simulink model "RT_TestMV_ATS"  (R2015b)
settings: Solver=FixedStepDiscrete  StartTime=0.0  StopTime=44.14  FixedStep=samplePeriod  RelTol=1e-3
PreLoadFcn:
  | initialize;
  | scramInitialize;
  | KR_alpha;
  | Discrete_Compensator;
  | ATS_setup
values from neighbouring files (symbols this model uses):
  a_ratio = K2/K1    (= 0.214196975539)    [KR_alpha.m]
  a_sub = ones(DOF_sub,1)    [KR_alpha.m]
  A_sub = (dt*alpha1_sub)/(Msub-Msub*alpha3_sub)    [KR_alpha.m]
  a_sup = ones(DOF_sup,1)    [KR_alpha.m]
  A_sup = (dt*alpha1_sup)/(Msup-Msup*alpha3_sup)    [KR_alpha.m]
  a_vector = ones(DOF,1)    [KR_alpha.m]
  alpha_f_sub = rho_inf_sub/(rho_inf_sub+1)    (= 0.5)    [KR_alpha.m]
  alpha_f_sup = rho_inf_sup/(rho_inf_sup+1)    (= 0.5)    [KR_alpha.m]
  B_sub = ((1/dt)*Msub*alpha3_sub)/alpha1_sub    [KR_alpha.m]
  B_sup = ((1/dt)*Msup*alpha3_sup)/alpha1_sup    [KR_alpha.m]
  controlPeriod = 1/2048    (= 0.00048828125)    [initialize.m]
  Csub = betaKinit*Ksub    [KR_alpha.m]
  Csup = (2*0.01/w1)*Ksup    (= 0.00743030767319)    [KR_alpha.m]
  D_sub = inv(alpha1_sub)/dt    [KR_alpha.m]
  D_sup = inv(alpha1_sup)/dt    [KR_alpha.m]
  dt = samplePeriod    [KR_alpha.m]
  forc_fbk_gain = 1.00    (= 1)    [KR_alpha.m]
  g = 386.089    [KR_alpha.m]
  gamma_sub = 0.5-alpha_m_sub+alpha_f_sub    (= 0.5)    [KR_alpha.m]
  gamma_sup = 0.5-alpha_m_sup+alpha_f_sup    (= 0.5)    [KR_alpha.m]
  K1 = 4.6686*K2    (= 9.3372)    [KR_alpha.m]
  K2 = 0.5*4    (= 2)    [KR_alpha.m]
  Ksub = Kstory    [KR_alpha.m]
  Msub = (0.88585/(56/450))*Mstory    (= 1.03248862309)    [KR_alpha.m]
  Msup = Mstory    (= 0.145044277356)    [KR_alpha.m]
  nAct = 4    [initialize.m]
  nDout = 4    [initialize.m]
  onesec = ceil(1/samplePeriod)    [Discrete_Compensator.m]
  samplePeriod = controlPeriod/upsampleFactor    (= 0.00048828125)    [initialize.m]
  scale_GM = 1.50    (= 1.5)    [KR_alpha.m]
  uy = 0.85    [KR_alpha.m]
undefined symbols (not defined in the file or in its folder): lhpNode, MRC, Nl, P_range, sample, SN, stsNode, Threshold, Zden, Znum
undefined symbols (not defined in the file): HybridCtrlParameters, Par
libraries: simulink x34, slrtlib x8, xpcsystranlib x5
(part 2 of 2)

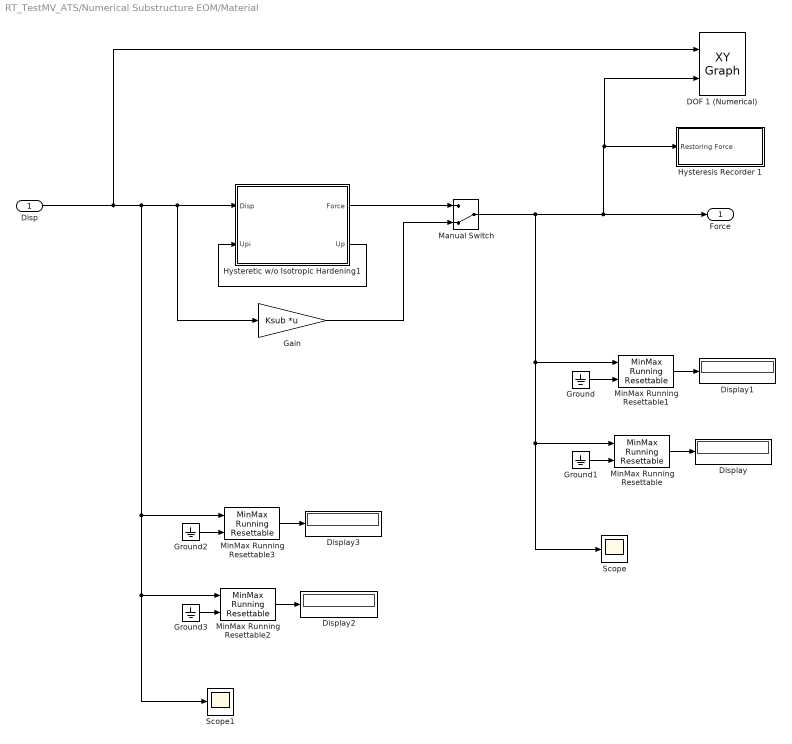
== system RT_TestMV_ATS/Numerical Substructure EOM/Material ==
  Disp : Inport
  DOF 1 (Numerical) : simulink/Sinks/XY Graph  xmin=-1  xmax=1  ymin=-35  ymax=35  st=-1
  Display{,1..3} (4 alike) : Display
  Gain : Gain  Gain=Ksub  Multiplication=Matrix(K*u) (u vector)
  Ground{,1..3} (4 alike) : Ground
  Hysteresis Recorder 1 : Subsystem
  Hysteretic w/o Isotropic Hardening1 : Subsystem
  Manual Switch : ManualSwitch  CurrentSetting=0
  MinMax Running Resettable : simulink/Math Operations/MinMax Running Resettable  Function=max  vinit=0.0
  MinMax Running Resettable1 : simulink/Math Operations/MinMax Running Resettable  Function=min  vinit=0.0
  MinMax Running Resettable2 : simulink/Math Operations/MinMax Running Resettable  Function=max  vinit=0.0
  MinMax Running Resettable3 : simulink/Math Operations/MinMax Running Resettable  Function=min  vinit=0.0
  Scope : Scope
  Scope1 : Scope
  Force : Outport
  wires:
  Hysteretic w/o Isotropic Hardening1/2(Up) -> Hysteretic w/o Isotropic Hardening1/2(Upi)
  Hysteretic w/o Isotropic Hardening1/1(Force) -> Manual Switch/1
  Gain/1 -> Manual Switch/2
  Ground2/1 -> MinMax Running Resettable3/2
  Ground/1 -> MinMax Running Resettable1/2
  MinMax Running Resettable2/1 -> Display2/1
  Manual Switch/1 -> MinMax Running Resettable1/1, MinMax Running Resettable/1, Scope/1, DOF 1 (Numerical)/2, Hysteresis Recorder 1/1(Restoring Force), Force/1
  MinMax Running Resettable3/1 -> Display3/1
  MinMax Running Resettable1/1 -> Display1/1
  Ground1/1 -> MinMax Running Resettable/2
  Disp/1 -> MinMax Running Resettable3/1, MinMax Running Resettable2/1, Scope1/1, Gain/1, Hysteretic w/o Isotropic Hardening1/1(Disp), DOF 1 (Numerical)/1
  Ground3/1 -> MinMax Running Resettable2/2
  MinMax Running Resettable/1 -> Display/1

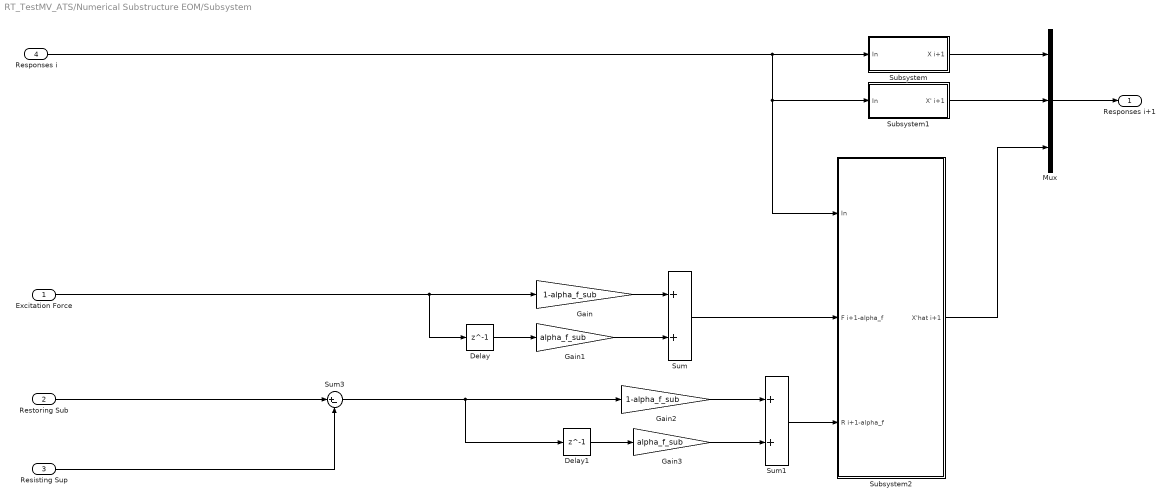
== system RT_TestMV_ATS/Numerical Substructure EOM/Subsystem ==
  Excitation Force : Inport
  Restoring Sub : Inport  Port=2
  Resisting Sup : Inport  Port=3
  Responses i : Inport  Port=4
  Delay : Delay  DelayLength=1
  Delay1 : Delay  DelayLength=1
  Gain : Gain  Gain=1-alpha_f_sub
  Gain1 : Gain  Gain=alpha_f_sub
  Gain2 : Gain  Gain=1-alpha_f_sub
  Gain3 : Gain  Gain=alpha_f_sub
  Mux : Mux  Inputs=3
  Subsystem : Subsystem
  Subsystem1 : Subsystem
  Subsystem2 : Subsystem
  Sum : Sum
  Sum1 : Sum
  Sum3 : Sum  Inputs=|+-
  Responses i+1 : Outport
  wires:
  Excitation Force/1 -> Delay/1, Gain/1
  Delay/1 -> Gain1/1
  Gain/1 -> Sum/1
  Gain1/1 -> Sum/2
  Sum/1 -> Subsystem2/2(F i+1-alpha_f)
  Mux/1 -> Responses i+1/1
  Subsystem1/1(X' i+1) -> Mux/2
  Subsystem/1(X i+1) -> Mux/1
  Subsystem2/1(X'hat i+1) -> Mux/3
  Delay1/1 -> Gain3/1
  Gain2/1 -> Sum1/1
  Gain3/1 -> Sum1/2
  Sum1/1 -> Subsystem2/3(R i+1-alpha_f)
  Responses i/1 -> Subsystem2/1(In), Subsystem1/1(In), Subsystem/1(In)
  Sum3/1 -> Delay1/1, Gain2/1
  Restoring Sub/1 -> Sum3/1
  Resisting Sup/1 -> Sum3/2

== system RT_TestMV_ATS/Offset/If Action ==
  In1 : Inport
  Action Port : ActionPort  PropagateVarSize=During execution  ActionType=then
  Data Store Read : DataStoreRead  DataStoreName=x0  SampleTime=controlPeriod
  Data Store Write : DataStoreWrite  DataStoreName=x0
  Gain : Gain  Gain=1/nOffset  SaturateOnIntegerOverflow=on  OutDataTypeStr=Inherit: Same as input  ParamDataTypeStr=Inherit: Same as input
  Sum : Sum  Inputs=|++  SaturateOnIntegerOverflow=on  InputSameDT=on  OutDataTypeStr=Inherit: Same as first input
  wires:
  Data Store Read/1 -> Sum/2
  Sum/1 -> Data Store Write/1
  Gain/1 -> Sum/1
  In1/1 -> Gain/1

== system RT_TestMV_ATS/Offset1/If Action ==
  In1 : Inport
  Action Port : ActionPort  PropagateVarSize=During execution  ActionType=then
  Data Store Read : DataStoreRead  DataStoreName=x0  SampleTime=controlPeriod
  Data Store Write : DataStoreWrite  DataStoreName=x0
  Gain : Gain  Gain=1/nOffset  SaturateOnIntegerOverflow=on  OutDataTypeStr=Inherit: Same as input  ParamDataTypeStr=Inherit: Same as input
  Sum : Sum  Inputs=|++  SaturateOnIntegerOverflow=on  InputSameDT=on  OutDataTypeStr=Inherit: Same as first input
  wires:
  Data Store Read/1 -> Sum/2
  Sum/1 -> Data Store Write/1
  Gain/1 -> Sum/1
  In1/1 -> Gain/1

== system RT_TestMV_ATS/Offset2/If Action ==
  In1 : Inport
  Action Port : ActionPort  PropagateVarSize=During execution  ActionType=then
  Data Store Read : DataStoreRead  DataStoreName=x0  SampleTime=controlPeriod
  Data Store Write : DataStoreWrite  DataStoreName=x0
  Gain : Gain  Gain=1/nOffset  SaturateOnIntegerOverflow=on  OutDataTypeStr=Inherit: Same as input  ParamDataTypeStr=Inherit: Same as input
  Sum : Sum  Inputs=|++  SaturateOnIntegerOverflow=on  InputSameDT=on  OutDataTypeStr=Inherit: Same as first input
  wires:
  Data Store Read/1 -> Sum/2
  Sum/1 -> Data Store Write/1
  Gain/1 -> Sum/1
  In1/1 -> Gain/1

== system RT_TestMV_ATS/Offset3/If Action ==
  In1 : Inport
  Action Port : ActionPort  PropagateVarSize=During execution  ActionType=then
  Data Store Read : DataStoreRead  DataStoreName=x0  SampleTime=controlPeriod
  Data Store Write : DataStoreWrite  DataStoreName=x0
  Gain : Gain  Gain=1/nOffset  SaturateOnIntegerOverflow=on  OutDataTypeStr=Inherit: Same as input  ParamDataTypeStr=Inherit: Same as input
  Sum : Sum  Inputs=|++  SaturateOnIntegerOverflow=on  InputSameDT=on  OutDataTypeStr=Inherit: Same as first input
  wires:
  Data Store Read/1 -> Sum/2
  Sum/1 -> Data Store Write/1
  Gain/1 -> Sum/1
  In1/1 -> Gain/1

== system RT_TestMV_ATS/Offset4/If Action ==
  In1 : Inport
  Action Port : ActionPort  PropagateVarSize=During execution  ActionType=then
  Data Store Read : DataStoreRead  DataStoreName=x0  SampleTime=controlPeriod
  Data Store Write : DataStoreWrite  DataStoreName=x0
  Gain : Gain  Gain=1/nOffset  SaturateOnIntegerOverflow=on  OutDataTypeStr=Inherit: Same as input  ParamDataTypeStr=Inherit: Same as input
  Sum : Sum  Inputs=|++  SaturateOnIntegerOverflow=on  InputSameDT=on  OutDataTypeStr=Inherit: Same as first input
  wires:
  Data Store Read/1 -> Sum/2
  Sum/1 -> Data Store Write/1
  Gain/1 -> Sum/1
  In1/1 -> Gain/1

== system RT_TestMV_ATS/Offset5/If Action ==
  In1 : Inport
  Action Port : ActionPort  PropagateVarSize=During execution  ActionType=then
  Data Store Read : DataStoreRead  DataStoreName=x0  SampleTime=controlPeriod
  Data Store Write : DataStoreWrite  DataStoreName=x0
  Gain : Gain  Gain=1/nOffset  SaturateOnIntegerOverflow=on  OutDataTypeStr=Inherit: Same as input  ParamDataTypeStr=Inherit: Same as input
  Sum : Sum  Inputs=|++  SaturateOnIntegerOverflow=on  InputSameDT=on  OutDataTypeStr=Inherit: Same as first input
  wires:
  Data Store Read/1 -> Sum/2
  Sum/1 -> Data Store Write/1
  Gain/1 -> Sum/1
  In1/1 -> Gain/1

== system RT_TestMV_ATS/Offset6/If Action ==
  In1 : Inport
  Action Port : ActionPort  PropagateVarSize=During execution  ActionType=then
  Data Store Read : DataStoreRead  DataStoreName=x0  SampleTime=controlPeriod
  Data Store Write : DataStoreWrite  DataStoreName=x0
  Gain : Gain  Gain=1/nOffset  SaturateOnIntegerOverflow=on  OutDataTypeStr=Inherit: Same as input  ParamDataTypeStr=Inherit: Same as input
  Sum : Sum  Inputs=|++  SaturateOnIntegerOverflow=on  InputSameDT=on  OutDataTypeStr=Inherit: Same as first input
  wires:
  Data Store Read/1 -> Sum/2
  Sum/1 -> Data Store Write/1
  Gain/1 -> Sum/1
  In1/1 -> Gain/1

== system RT_TestMV_ATS/Offset7/If Action ==
  In1 : Inport
  Action Port : ActionPort  PropagateVarSize=During execution  ActionType=then
  Data Store Read : DataStoreRead  DataStoreName=x0  SampleTime=controlPeriod
  Data Store Write : DataStoreWrite  DataStoreName=x0
  Gain : Gain  Gain=1/nOffset  SaturateOnIntegerOverflow=on  OutDataTypeStr=Inherit: Same as input  ParamDataTypeStr=Inherit: Same as input
  Sum : Sum  Inputs=|++  SaturateOnIntegerOverflow=on  InputSameDT=on  OutDataTypeStr=Inherit: Same as first input
  wires:
  Data Store Read/1 -> Sum/2
  Sum/1 -> Data Store Write/1
  Gain/1 -> Sum/1
  In1/1 -> Gain/1

== system RT_TestMV_ATS/Responses Recorder/Drifts ==
  In1 : Inport
  Demux : Demux  Outputs=2
  Sum5 : Sum  Inputs=-|+||
  Drift DOF 1 : Outport
  Drift DOF 2 : Outport  Port=2
  wires:
  In1/1 -> Demux/1
  Demux/2 -> Sum5/2
  Demux/1 -> Sum5/1, Drift DOF 1/1
  Sum5/1 -> Drift DOF 2/1

== system RT_TestMV_ATS/Base Shear/Offset1/If Action ==
  In1 : Inport
  Action Port : ActionPort  PropagateVarSize=During execution  ActionType=then
  Data Store Read : DataStoreRead  DataStoreName=x0  SampleTime=controlPeriod
  Data Store Write : DataStoreWrite  DataStoreName=x0
  Gain : Gain  Gain=1/nOffset  SaturateOnIntegerOverflow=on  OutDataTypeStr=Inherit: Same as input  ParamDataTypeStr=Inherit: Same as input
  Sum : Sum  Inputs=|++  SaturateOnIntegerOverflow=on  InputSameDT=on  OutDataTypeStr=Inherit: Same as first input
  wires:
  Data Store Read/1 -> Sum/2
  Sum/1 -> Data Store Write/1
  Gain/1 -> Sum/1
  In1/1 -> Gain/1

== system RT_TestMV_ATS/Base Shear/Offset2/If Action ==
  In1 : Inport
  Action Port : ActionPort  PropagateVarSize=During execution  ActionType=then
  Data Store Read : DataStoreRead  DataStoreName=x0  SampleTime=controlPeriod
  Data Store Write : DataStoreWrite  DataStoreName=x0
  Gain : Gain  Gain=1/nOffset  SaturateOnIntegerOverflow=on  OutDataTypeStr=Inherit: Same as input  ParamDataTypeStr=Inherit: Same as input
  Sum : Sum  Inputs=|++  SaturateOnIntegerOverflow=on  InputSameDT=on  OutDataTypeStr=Inherit: Same as first input
  wires:
  Data Store Read/1 -> Sum/2
  Sum/1 -> Data Store Write/1
  Gain/1 -> Sum/1
  In1/1 -> Gain/1

== system RT_TestMV_ATS/Base Shear/Offset3/If Action ==
  In1 : Inport
  Action Port : ActionPort  PropagateVarSize=During execution  ActionType=then
  Data Store Read : DataStoreRead  DataStoreName=x0  SampleTime=controlPeriod
  Data Store Write : DataStoreWrite  DataStoreName=x0
  Gain : Gain  Gain=1/nOffset  SaturateOnIntegerOverflow=on  OutDataTypeStr=Inherit: Same as input  ParamDataTypeStr=Inherit: Same as input
  Sum : Sum  Inputs=|++  SaturateOnIntegerOverflow=on  InputSameDT=on  OutDataTypeStr=Inherit: Same as first input
  wires:
  Data Store Read/1 -> Sum/2
  Sum/1 -> Data Store Write/1
  Gain/1 -> Sum/1
  In1/1 -> Gain/1

== system RT_TestMV_ATS/Base Shear/Offset4/If Action ==
  In1 : Inport
  Action Port : ActionPort  PropagateVarSize=During execution  ActionType=then
  Data Store Read : DataStoreRead  DataStoreName=x0  SampleTime=controlPeriod
  Data Store Write : DataStoreWrite  DataStoreName=x0
  Gain : Gain  Gain=1/nOffset  SaturateOnIntegerOverflow=on  OutDataTypeStr=Inherit: Same as input  ParamDataTypeStr=Inherit: Same as input
  Sum : Sum  Inputs=|++  SaturateOnIntegerOverflow=on  InputSameDT=on  OutDataTypeStr=Inherit: Same as first input
  wires:
  Data Store Read/1 -> Sum/2
  Sum/1 -> Data Store Write/1
  Gain/1 -> Sum/1
  In1/1 -> Gain/1

== system RT_TestMV_ATS/Experimental Superstructure EOM/Material/Hysteresis Recorder 1 ==
  Restoring Force : Inport
  To File2 : ToFile  Filename=Restoring_DOF2.mat  MatrixName=Restoring_DOF2
  wires:
  Restoring Force/1 -> To File2/1

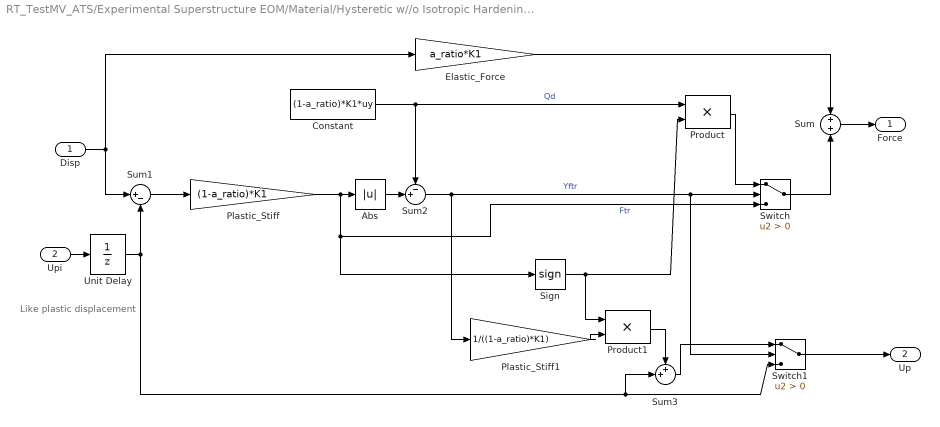
== system RT_TestMV_ATS/Experimental Superstructure EOM/Material/Hysteretic w//o Isotropic Hardening1 ==
  note: Like plastic displacement
  Disp : Inport
  Upi : Inport  Port=2
  Abs : Abs  SaturateOnIntegerOverflow=on
  Constant : Constant  Value=(1-a_ratio)*K1*uy
  Elastic_Force : Gain  Gain=a_ratio*K1  SaturateOnIntegerOverflow=on  OutDataTypeStr=Inherit: Same as input  ParamDataTypeStr=Inherit: Same as input
  Plastic_Stiff : Gain  Gain=(1-a_ratio)*K1  SaturateOnIntegerOverflow=on  OutDataTypeStr=Inherit: Same as input  ParamDataTypeStr=Inherit: Same as input
  Plastic_Stiff1 : Gain  Gain=1/((1-a_ratio)*K1)  SaturateOnIntegerOverflow=on  OutDataTypeStr=Inherit: Same as input  ParamDataTypeStr=Inherit: Same as input
  Product : Product  SaturateOnIntegerOverflow=on  OutDataTypeStr=Inherit: Same as first input
  Product1 : Product  SaturateOnIntegerOverflow=on  OutDataTypeStr=Inherit: Same as first input
  Sign : Signum
  Sum : Sum  Inputs=+|+  SaturateOnIntegerOverflow=on  InputSameDT=on  OutDataTypeStr=Inherit: Same as first input
  Sum1 : Sum  Inputs=|+-  SaturateOnIntegerOverflow=on
  Sum2 : Sum  Inputs=-+|  SaturateOnIntegerOverflow=on
  Sum3 : Sum  Inputs=++|  SaturateOnIntegerOverflow=on
  Switch : Switch  Criteria=u2 > Threshold  SaturateOnIntegerOverflow=on
  Switch1 : Switch  Criteria=u2 > Threshold  SaturateOnIntegerOverflow=on
  Unit Delay : UnitDelay  SampleTime=-1
  Force : Outport
  Up : Outport  Port=2
  wires:
  Elastic_Force/1 -> Sum/1
  Disp/1 -> Sum1/1, Elastic_Force/1
  Sum/1 -> Force/1
  Upi/1 -> Unit Delay/1
  Sum1/1 -> Plastic_Stiff/1
  Plastic_Stiff/1 -> Abs/1, Switch/3, Sign/1  "Ftr"
  Constant/1 -> Sum2/1, Product/1  "Qd"
  Sum2/1 -> Switch/2, Switch1/2, Plastic_Stiff1/1  "Yftr"
  Product/1 -> Switch/1
  Switch/1 -> Sum/2
  Switch1/1 -> Up/1
  Sum3/1 -> Switch1/1
  Product1/1 -> Sum3/1
  Plastic_Stiff1/1 -> Product1/2
  Unit Delay/1 -> Sum1/2, Sum3/2, Switch1/3
  Sign/1 -> Product1/1, Product/2
  Abs/1 -> Sum2/2

== system RT_TestMV_ATS/Experimental Superstructure EOM/Subsystem/Subsystem ==
  In : Inport
  Demux : Demux  Outputs=3
  Gain : Gain  Gain=dt
  Gain1 : Gain  Gain=(0.5+gamma_sup)*dt
  Sum1 : Sum  Inputs=+++
  X i+1 : Outport
  wires:
  In/1 -> Demux/1
  Demux/3 -> Gain1/1
  Demux/2 -> Gain/1
  Demux/1 -> Sum1/1
  Gain/1 -> Sum1/2
  Gain1/1 -> Sum1/3
  Sum1/1 -> X i+1/1

== system RT_TestMV_ATS/Experimental Superstructure EOM/Subsystem/Subsystem1 ==
  In : Inport
  Demux : Demux  Outputs=3
  Sum : Sum  Inputs=|++
  Terminator : Terminator
  X' i+1 : Outport
  wires:
  In/1 -> Demux/1
  Sum/1 -> X' i+1/1
  Demux/3 -> Sum/2
  Demux/2 -> Sum/1
  Demux/1 -> Terminator/1

== system RT_TestMV_ATS/Experimental Superstructure EOM/Subsystem/Subsystem2 ==
  In : Inport
  F i+1-alpha_f : Inport  Port=2
  R i+1-alpha_f : Inport  Port=3
  Demux : Demux  Outputs=3
  Gain : Gain  Gain=B_sup  Multiplication=Matrix(K*u) (u vector)
  Gain1 : Gain  Gain=1-alpha_f_sup
  Gain2 : Gain  Gain=Csup  Multiplication=Matrix(K*u) (u vector)
  Gain3 : Gain  Gain=A_sup  Multiplication=Matrix(K*u) (u vector)
  Sum : Sum  Inputs=+---
  Sum1 : Sum  Inputs=|++
  Terminator : Terminator
  X'hat i+1 : Outport
  wires:
  In/1 -> Demux/1
  Demux/3 -> Gain/1, Gain1/1
  Gain/1 -> Sum/4
  Demux/2 -> Sum1/1
  Sum1/1 -> Gain2/1
  Gain1/1 -> Sum1/2
  Gain2/1 -> Sum/2
  F i+1-alpha_f/1 -> Sum/1
  R i+1-alpha_f/1 -> Sum/3
  Sum/1 -> Gain3/1
  Gain3/1 -> X'hat i+1/1
  Demux/1 -> Terminator/1

== system RT_TestMV_ATS/Numerical Substructure EOM/Material/Hysteresis Recorder 1 ==
  Restoring Force : Inport
  To File2 : ToFile  Filename=Restoring_DOF1.mat  MatrixName=Restoring_DOF1
  wires:
  Restoring Force/1 -> To File2/1

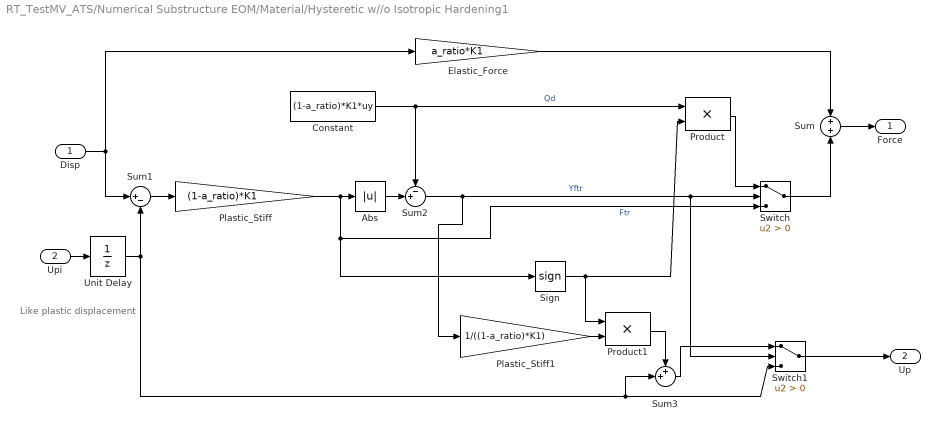
== system RT_TestMV_ATS/Numerical Substructure EOM/Material/Hysteretic w//o Isotropic Hardening1 ==
  note: Like plastic displacement
  Disp : Inport
  Upi : Inport  Port=2
  Abs : Abs  SaturateOnIntegerOverflow=on
  Constant : Constant  Value=(1-a_ratio)*K1*uy
  Elastic_Force : Gain  Gain=a_ratio*K1  SaturateOnIntegerOverflow=on  OutDataTypeStr=Inherit: Same as input  ParamDataTypeStr=Inherit: Same as input
  Plastic_Stiff : Gain  Gain=(1-a_ratio)*K1  SaturateOnIntegerOverflow=on  OutDataTypeStr=Inherit: Same as input  ParamDataTypeStr=Inherit: Same as input
  Plastic_Stiff1 : Gain  Gain=1/((1-a_ratio)*K1)  SaturateOnIntegerOverflow=on  OutDataTypeStr=Inherit: Same as input  ParamDataTypeStr=Inherit: Same as input
  Product : Product  SaturateOnIntegerOverflow=on  OutDataTypeStr=Inherit: Same as first input
  Product1 : Product  SaturateOnIntegerOverflow=on  OutDataTypeStr=Inherit: Same as first input
  Sign : Signum
  Sum : Sum  Inputs=+|+  SaturateOnIntegerOverflow=on  InputSameDT=on  OutDataTypeStr=Inherit: Same as first input
  Sum1 : Sum  Inputs=|+-  SaturateOnIntegerOverflow=on
  Sum2 : Sum  Inputs=-+|  SaturateOnIntegerOverflow=on
  Sum3 : Sum  Inputs=++|  SaturateOnIntegerOverflow=on
  Switch : Switch  Criteria=u2 > Threshold  SaturateOnIntegerOverflow=on
  Switch1 : Switch  Criteria=u2 > Threshold  SaturateOnIntegerOverflow=on
  Unit Delay : UnitDelay  SampleTime=-1
  Force : Outport
  Up : Outport  Port=2
  wires:
  Elastic_Force/1 -> Sum/1
  Disp/1 -> Sum1/1, Elastic_Force/1
  Sum/1 -> Force/1
  Upi/1 -> Unit Delay/1
  Sum1/1 -> Plastic_Stiff/1
  Plastic_Stiff/1 -> Abs/1, Switch/3, Sign/1  "Ftr"
  Constant/1 -> Sum2/1, Product/1  "Qd"
  Sum2/1 -> Switch/2, Switch1/2, Plastic_Stiff1/1  "Yftr"
  Product/1 -> Switch/1
  Switch/1 -> Sum/2
  Switch1/1 -> Up/1
  Sum3/1 -> Switch1/1
  Product1/1 -> Sum3/1
  Plastic_Stiff1/1 -> Product1/2
  Unit Delay/1 -> Sum1/2, Sum3/2, Switch1/3
  Sign/1 -> Product1/1, Product/2
  Abs/1 -> Sum2/2

== system RT_TestMV_ATS/Numerical Substructure EOM/Subsystem/Subsystem ==
  In : Inport
  Demux : Demux  Outputs=3
  Gain : Gain  Gain=dt
  Gain1 : Gain  Gain=(0.5+gamma_sub)*dt
  Sum1 : Sum  Inputs=+++
  X i+1 : Outport
  wires:
  In/1 -> Demux/1
  Demux/3 -> Gain1/1
  Demux/2 -> Gain/1
  Demux/1 -> Sum1/1
  Gain/1 -> Sum1/2
  Gain1/1 -> Sum1/3
  Sum1/1 -> X i+1/1

== system RT_TestMV_ATS/Numerical Substructure EOM/Subsystem/Subsystem1 ==
  In : Inport
  Demux : Demux  Outputs=3
  Sum : Sum  Inputs=|++
  Terminator : Terminator
  X' i+1 : Outport
  wires:
  In/1 -> Demux/1
  Sum/1 -> X' i+1/1
  Demux/3 -> Sum/2
  Demux/2 -> Sum/1
  Demux/1 -> Terminator/1

== system RT_TestMV_ATS/Numerical Substructure EOM/Subsystem/Subsystem2 ==
  In : Inport
  F i+1-alpha_f : Inport  Port=2
  R i+1-alpha_f : Inport  Port=3
  Demux : Demux  Outputs=3
  Gain : Gain  Gain=B_sub  Multiplication=Matrix(K*u) (u vector)
  Gain1 : Gain  Gain=1-alpha_f_sub
  Gain2 : Gain  Gain=Csub  Multiplication=Matrix(K*u) (u vector)
  Gain3 : Gain  Gain=A_sub  Multiplication=Matrix(K*u) (u vector)
  Sum : Sum  Inputs=+---
  Sum1 : Sum  Inputs=|++
  Terminator : Terminator
  X'hat i+1 : Outport
  wires:
  In/1 -> Demux/1
  Demux/3 -> Gain/1, Gain1/1
  Gain/1 -> Sum/4
  Demux/2 -> Sum1/1
  Sum1/1 -> Gain2/1
  Gain1/1 -> Sum1/2
  Gain2/1 -> Sum/2
  F i+1-alpha_f/1 -> Sum/1
  R i+1-alpha_f/1 -> Sum/3
  Sum/1 -> Gain3/1
  Gain3/1 -> X'hat i+1/1
  Demux/1 -> Terminator/1

== matlab function RT_TestMV_ATS/ATS compensator/calculate optimal coefficients ==
  data: threshold input; par input; p_range input; MRC input; X1 input; apar output; X2 input; X3 input; Y input; dm input; prev_par input; triggeri input
function apar = fcn(threshold,par,p_range,MRC,X1,X2,X3,Y,dm,prev_par,triggeri)
%#codegen
%triggero=triggeri;
apar = [par; triggeri];

if( abs( dm ) > threshold || apar(4) )
    apar(4)=1;
    
    X = [X1 X2 X3];       
    
    temp=X\Y; 
    
    apar(1:3)=temp;
    
    if( isnan( apar(1) ) + isnan( apar(2) ) + isnan( apar(3) ) )
        apar=[par; triggeri];
    end
    
    
    % maximum change of rate
    if( abs(apar(1)-prev_par(1)) > MRC(1) )
        apar(1) = prev_par(1) + sign(apar(1)-prev_par(1))*MRC(1);
    end
    if( abs(apar(2)-prev_par(2)) > MRC(2) )
        apar(2) = prev_par(2) + sign(apar(2)-prev_par(2))*MRC(2);
    end
    if( abs(apar(3)-prev_par(3)) > MRC(3) )
        apar(3) = prev_par(3) + sign(apar(3)-prev_par(3))*MRC(3);
    end
    
    % limit of coefficients
    if( apar(1) < p_range(1,1) )
        apar(1) = p_range(1,1);
    end
    
    if( apar(1) > p_range(1,2) )
        apar(1) = p_range(1,2);
    end
    
    if( apar(2) < p_range(2,1) )
        apar(2) = p_range(2,1);
    end
    
    if( apar(2) > p_range(2,2) )
        apar(2) = p_range(2,2);
    end
    
    if( apar(3) < p_range(3,1) )
        apar(3) = p_range(3,1);
    end
    
    if( apar(3) > p_range(3,2) )
        apar(3) = p_range(3,2);
    end    
    
end

== matlab function RT_TestMV_ATS/ATS compensator/compensated actuator input disp. ==
  data: apar input; x input; xd input; x2d input; ut_pred output
function ut_pred = fcn(apar,x,xd,x2d)
%#codegen

ut_pred = apar(1)*x + apar(2)*xd + apar(3)*x2d;
